simulink model "forced_msd_uin"  (Simulink 7.8)
settings: Solver=ode4  StartTime=0.0  StopTime=time_span  RelTol=1e-3
undefined symbols (not defined in the file or in its folder): outstr, samp_time
settings Model: Creator=Kourosh Danai  LastModifiedBy=BionicBill
settings DataIOCC: TimeSaveName=t  OutputSaveName=y
settings DebuggingCC: AlgebraicLoopMsg=none  FcnCallInpInsideContextMsg=Use local settings  StrictBusMsg=Warning
settings SFSimCC: SimParseCustomCode=off

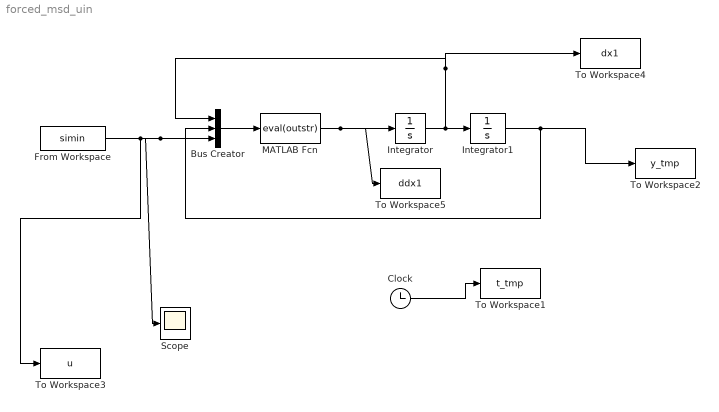
== system forced_msd_uin ==
  Bus Creator : BusCreator  Inputs=3
  Clock : Clock
  From Workspace : FromWorkspace  VariableName=simin  SampleTime=0
  Integrator : Integrator
  Integrator1 : Integrator
  MATLAB Fcn : MATLABFcn  MATLABFcn=eval(outstr)
  Scope : Scope
  To Workspace1 : ToWorkspace  VariableName=t_tmp  SampleTime=samp_time  SaveFormat=Array
  To Workspace2 : ToWorkspace  VariableName=y_tmp  SampleTime=samp_time  SaveFormat=Array
  To Workspace3 : ToWorkspace  VariableName=u  SampleTime=-1  SaveFormat=Array
  To Workspace4 : ToWorkspace  VariableName=dx1  SampleTime=samp_time  SaveFormat=Array
  To Workspace5 : ToWorkspace  VariableName=ddx1  SampleTime=samp_time  SaveFormat=Array
  wires:
  Integrator/1 -> Integrator1/1, Bus Creator/1, To Workspace4/1
  Bus Creator/1 -> MATLAB Fcn/1
  Clock/1 -> To Workspace1/1
  Integrator1/1 -> Bus Creator/2, To Workspace2/1
  MATLAB Fcn/1 -> Integrator/1, To Workspace5/1
  From Workspace/1 -> To Workspace3/1, Bus Creator/3, Scope/1
